simulink model "model"  (R2016a)
settings: Solver=FixedStepAuto  StartTime=0.0  StopTime=50  FixedStep=0.001  RelTol=1e-3
settings Model: Creator=Priscilla  LastModifiedBy=Priscilla

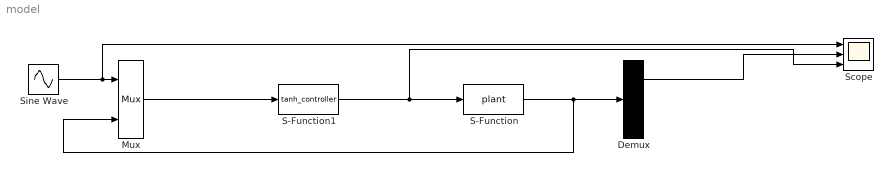
== system model ==
  Demux : Demux  Outputs=2
  Mux : Mux  Inputs=2
  S-Function : S-Function  FunctionName=plant  SFunctionDeploymentMode=off  EnableBusSupport=off
  S-Function1 : S-Function  FunctionName=tanh_controller  SFunctionDeploymentMode=off  EnableBusSupport=off
  Scope : Scope  NumInputPorts=3
  Sine Wave : Sin  SampleTime=0
  wires:
  S-Function/1 -> Mux/2, Demux/1
  S-Function1/1 -> Scope/3, S-Function/1
  Sine Wave/1 -> Scope/1, Mux/1
  Mux/1 -> S-Function1/1
  Demux/1 -> Scope/2
